simulink model "Inverse_Pendulum"  (R2025a)
settings: Solver=VariableStepAuto  StartTime=0.0  StopTime=50  RelTol=1e-3
values from neighbouring files (symbols this model uses):
  A = [ 0         0       1       0 ... (first row only)    [Inverse_Pendulum_parameters.m]    (also in Inverse_Pendulum_parameters_discrete.m; [LQG] Inverse_Pendulum_parameters.m; [LQR] Inverse_Pendulum_parameters.m)
  b = 0.00007892    (= 7.892e-05)    [Inverse_Pendulum_parameters.m]    (also in Inverse_Pendulum_parameters_discrete.m; [LQG] Inverse_Pendulum_parameters.m; [LQR] Inverse_Pendulum_parameters.m)
  B = [0;         0;          (J+m*l^2)*kt/(alp*Rm*r);        l*m*kt/(alp*Rm*r)]    [Inverse_Pendulum_parameters.m]    (also in Inverse_Pendulum_parameters_discrete.m; [LQG] Inverse_Pendulum_parameters.m; [LQR] Inverse_Pendulum_parameters.m)
  c = 0.63    [Inverse_Pendulum_parameters.m]    (also in Inverse_Pendulum_parameters_discrete.m; [LQG] Inverse_Pendulum_parameters.m; [LQR] Inverse_Pendulum_parameters.m)
  C = [1 0 0 0; 0 1 0 0]    [Inverse_Pendulum_parameters.m]    (also in Inverse_Pendulum_parameters_discrete.m; [LQG] Inverse_Pendulum_parameters.m)
  g = 9.81    [Inverse_Pendulum_parameters.m]    (also in Inverse_Pendulum_parameters_discrete.m; [LQG] Inverse_Pendulum_parameters.m; [LQR] Inverse_Pendulum_parameters.m)
  J = 0.0007176    [Inverse_Pendulum_parameters.m]    (also in Inverse_Pendulum_parameters_discrete.m = 0.000596; [LQG] Inverse_Pendulum_parameters.m; [LQR] Inverse_Pendulum_parameters.m)
  K = lqr(A,B,Q,R)    [Inverse_Pendulum_parameters.m]    (also in [LQG] Inverse_Pendulum_parameters.m; [LQR] Inverse_Pendulum_parameters.m)
  k_swing = 12    [Inverse_Pendulum_parameters.m]    (also in Inverse_Pendulum_parameters_discrete.m = 42; [LQG] Inverse_Pendulum_parameters.m; [LQR] Inverse_Pendulum_parameters.m)
  kb = 0.031    [Inverse_Pendulum_parameters.m]    (also in Inverse_Pendulum_parameters_discrete.m; [LQG] Inverse_Pendulum_parameters.m; [LQR] Inverse_Pendulum_parameters.m)
  Kk = lqe(A, G, C, Qn, Rn)    [Inverse_Pendulum_parameters.m]    (also in [LQG] Inverse_Pendulum_parameters.m)
  kt = 0.031    [Inverse_Pendulum_parameters.m]    (also in Inverse_Pendulum_parameters_discrete.m; [LQG] Inverse_Pendulum_parameters.m; [LQR] Inverse_Pendulum_parameters.m)
  l = 0.2    [Inverse_Pendulum_parameters.m]    (also in Inverse_Pendulum_parameters_discrete.m = 0.1; [LQG] Inverse_Pendulum_parameters.m; [LQR] Inverse_Pendulum_parameters.m)
  M = 0.136    [Inverse_Pendulum_parameters.m]    (also in Inverse_Pendulum_parameters_discrete.m = 0.1; [LQG] Inverse_Pendulum_parameters.m; [LQR] Inverse_Pendulum_parameters.m)
  m = 0.1    [Inverse_Pendulum_parameters.m]    (also in Inverse_Pendulum_parameters_discrete.m = 0.04467; [LQG] Inverse_Pendulum_parameters.m; [LQR] Inverse_Pendulum_parameters.m)
  r = 0.006    [Inverse_Pendulum_parameters.m]    (also in Inverse_Pendulum_parameters_discrete.m; [LQG] Inverse_Pendulum_parameters.m; [LQR] Inverse_Pendulum_parameters.m)
  Rm = 12.5    [Inverse_Pendulum_parameters.m]    (also in Inverse_Pendulum_parameters_discrete.m; [LQG] Inverse_Pendulum_parameters.m; [LQR] Inverse_Pendulum_parameters.m)
libraries: simulink x7
settings Model: Creator=ADMIN  LastModifiedBy=ADMIN
settings OptimizationCC: DefaultParameterBehavior=Inlined  EnhancedBackFolding=on  PassReuseOutputArgsAs=Individual arguments  ZeroExternalMemoryAtStartup=off  ZeroInternalMemoryAtStartup=off  OptimizeBlockOrder=speed  DifferentSizesBufferReuse=on  OptimizationCustomize=off  EfficientTunableParamExpr=on
settings DebuggingCC: ParameterTunabilityLossMsg=error
settings SFSimCC: MATLABDynamicMemAlloc=off
settings RTWCC: SystemTargetFile=ert.tlc  GenCodeOnly=on  TemplateMakefile=ert_default_tmf  Description=Embedded Coder
settings CodeAppCC: ForceParamTrailComments=on  IgnoreCustomStorageClasses=off  OperatorAnnotations=on  SimulinkDataObjDesc=on  SFDataObjDesc=on  InsertBlockDesc=on
settings ERTTargetCC: ExtModeTransport=0.0  ExtModeStaticAlloc=off  ExtModeMexFile=ext_comm  ExtModeIntrfLevel=Level1  ERTCustomFileTemplate=example_file_process.tlc  TargetLangStandard=C99 (ISO)  GenerateSampleERTMain=on

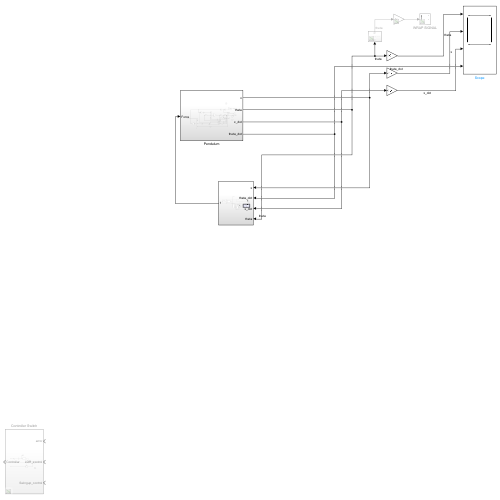
[thumbnail: Simulink's stored preview of the top-level diagram]
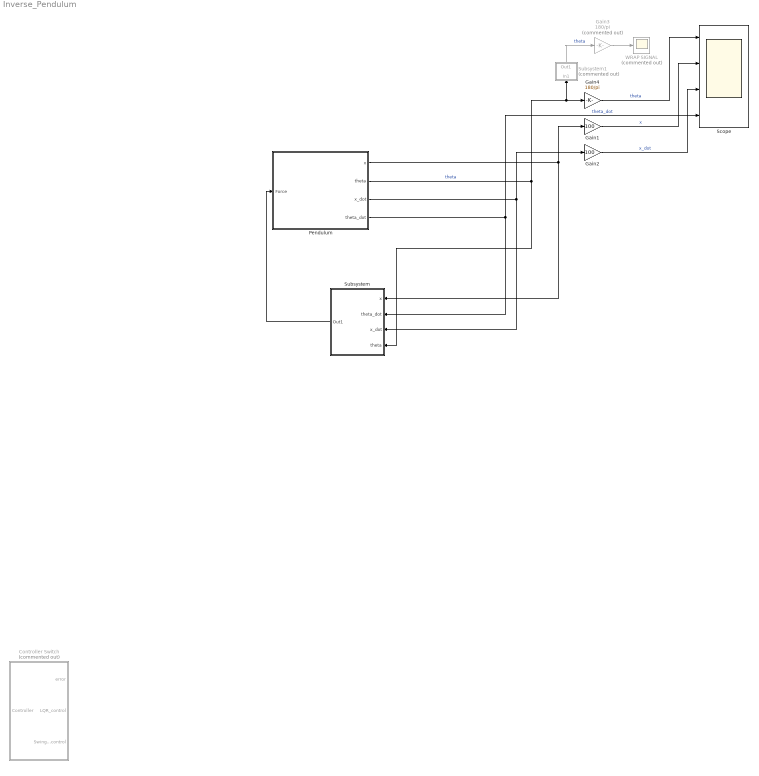
== system Inverse_Pendulum ==
  Controller Switch : Subsystem  Commented=on
  Gain1 : Gain  Gain=100
  Gain2 : Gain  Gain=100
  Gain3 : Gain  Commented=on  Gain=180/pi
  Gain4 : Gain  Gain=180/pi
  Pendulum : Subsystem
  Scope : Scope  NumInputPorts=4
      settings: ActiveDisplayYMinimum=-181.08264575614339  ActiveDisplayYMaximum=178.95893192046651
  Subsystem : Subsystem
  Subsystem1 : Subsystem  Commented=on
  WRAP SIGNAL : Scope  Commented=on
      settings: ActiveDisplayYMinimum=-145.61857492657683  ActiveDisplayYMaximum=445.48596723603623  DataLoggingVariableName=ScopeData3
  wires:
  Pendulum/1(x) -> Gain1/1, Subsystem/1(x)
  Pendulum/3(x_dot) -> Gain2/1, Subsystem/3(x_dot)
  Pendulum/4(theta_dot) -> Scope/4, Subsystem/2(theta_dot)  "theta_dot"
  Gain1/1 -> Scope/2  "x"
  Gain2/1 -> Scope/3  "x_dot"
  Pendulum/2(theta) -> Subsystem/4(theta), Subsystem1/1(In1), Gain4/1  "theta"
  Gain3/1 -> WRAP SIGNAL/1
  Subsystem1/1(Out1) -> Gain3/1  "theta"
  Gain4/1 -> Scope/1  "theta"
  Subsystem/1(Out1) -> Pendulum/1(Force)

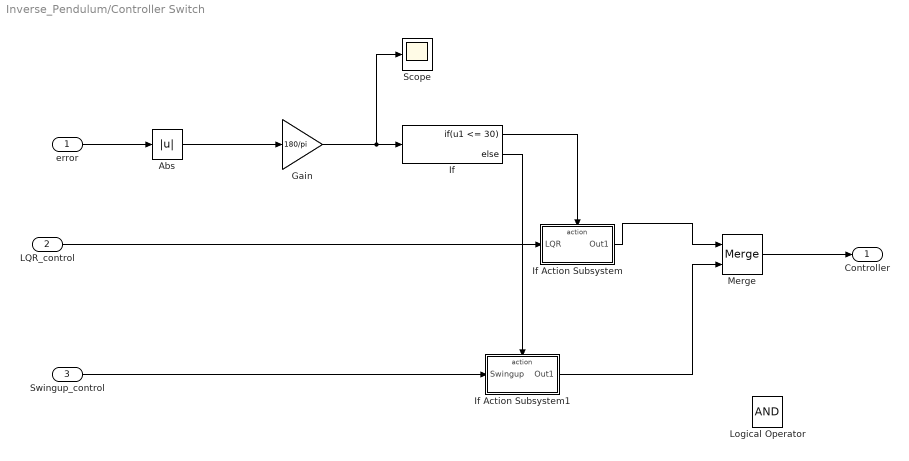
== system Inverse_Pendulum/Controller Switch ==
  error : Inport
  LQR_control : Inport  Port=2
  Swingup_control : Inport  Port=3
  Abs : Abs  SaturateOnIntegerOverflow=off
  Gain : Gain  Gain=180/pi
  If : If  IfExpression=u1 <= 30
  If Action Subsystem : Subsystem  TreatAsAtomicUnit=on
  If Action Subsystem1 : Subsystem  TreatAsAtomicUnit=on
  Logical Operator : Logic  AllPortsSameDT=off  OutDataTypeStr=boolean
  Merge : Merge
  Scope : Scope
      settings: ActiveDisplayYMinimum=-128.20702639105355  ActiveDisplayYMaximum=233.38136313352607  DataLoggingVariableName=ScopeData4
  Controller : Outport
  wires:
  error/1 -> Abs/1
  Abs/1 -> Gain/1
  Gain/1 -> Scope/1, If/1
  If/1 -> If Action Subsystem/Action
  LQR_control/1 -> If Action Subsystem/1(LQR)
  If/2 -> If Action Subsystem1/Action
  Swingup_control/1 -> If Action Subsystem1/1(Swingup)
  If Action Subsystem/1(Out1) -> Merge/1
  If Action Subsystem1/1(Out1) -> Merge/2
  Merge/1 -> Controller/1

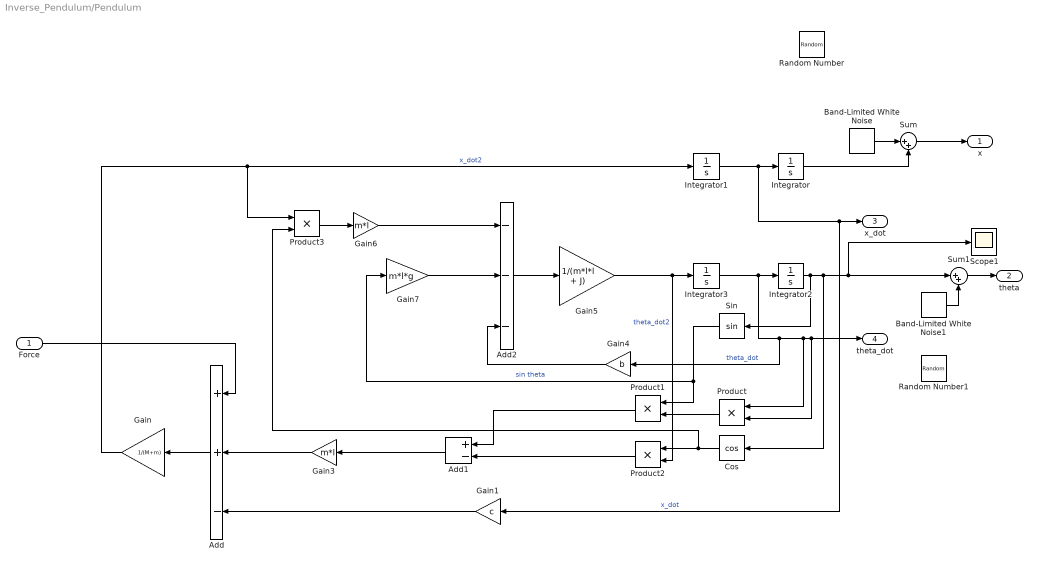
== system Inverse_Pendulum/Pendulum ==
  Force : Inport
  Add : Sum  Inputs=++-
  Add1 : Sum  Inputs=+-
  Add2 : Sum  Inputs=---
  Band-Limited White Noise : simulink/Sources/Band-Limited White Noise  Cov=[0.000001]  Ts=0.1  seed=[23341]
  Band-Limited White Noise1 : simulink/Sources/Band-Limited White Noise  Cov=[0.000001]  Ts=0.1  seed=[23341]
  Cos : Trigonometry  Operator=cos
  Gain : Gain  Gain=1/(M+m)
  Gain1 : Gain  Gain=c
  Gain3 : Gain  Gain=m*l
  Gain4 : Gain  Gain=b
  Gain5 : Gain  Gain=1/(m*l*l + J)
  Gain6 : Gain  Gain=m*l
  Gain7 : Gain  Gain=m*l*g
  Integrator{,1..3} (4 alike) : Integrator
  Product{,1..3} (4 alike) : Product
  Random Number : RandomNumber  Variance=0.001  SampleTime=0.1
  Random Number1 : RandomNumber  Variance=0.0001  SampleTime=0.1
  Scope1 : Scope
      settings: ActiveDisplayYMinimum=-24.198967580601451  ActiveDisplayYMaximum=45.388514798043275  DataLoggingVariableName=ScopeData2
  Sin : Trigonometry
  Sum : Sum  Inputs=|++
  Sum1 : Sum  Inputs=|++
  x : Outport
  theta : Outport  Port=2
  x_dot : Outport  Port=3
  theta_dot : Outport  Port=4
  wires:
  Gain3/1 -> Add/2
  Integrator/1 -> Sum/2
  Integrator1/1 -> Gain1/1, x_dot/1, Integrator/1  "x_dot"
  Product/1 -> Product1/2
  Force/1 -> Add/1
  Product1/1 -> Add1/1
  Sin/1 -> Gain7/1, Product1/1  "sin theta"
  Gain6/1 -> Add2/1
  Add2/1 -> Gain5/1
  Integrator3/1 -> theta_dot/1, Product/2, Product/1, Gain4/1, Integrator2/1  "theta_dot"
  Gain5/1 -> Product2/2, Integrator3/1  "theta_dot2"
  Integrator2/1 -> Cos/1, Sum1/1, Scope1/1, Sin/1
  Add/1 -> Gain/1
  Gain/1 -> Product3/1, Integrator1/1  "x_dot2"
  Gain7/1 -> Add2/2
  Cos/1 -> Product3/2, Product2/1
  Product3/1 -> Gain6/1
  Gain4/1 -> Add2/3
  Product2/1 -> Add1/2
  Add1/1 -> Gain3/1
  Gain1/1 -> Add/3
  Sum/1 -> x/1
  Sum1/1 -> theta/1
  Band-Limited White Noise/1 -> Sum/1
  Band-Limited White Noise1/1 -> Sum1/2

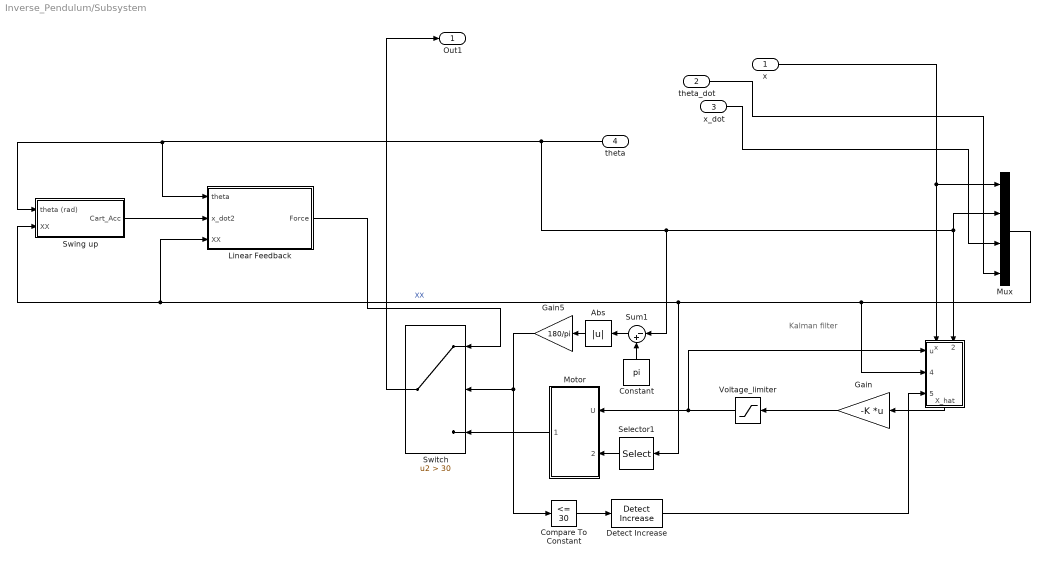
== system Inverse_Pendulum/Subsystem ==
  note: Kalman filter
  x : Inport
  theta_dot : Inport  Port=2
  x_dot : Inport  Port=3
  theta : Inport  Port=4
  " " : Subsystem
      settings: PortSchema="{\"entries\":[{\"content\":{\"sides\":[{\"content\":{\"connectorIds\":[\"In1\",\"In2\"]},\"type\":\"ConnectorPlacement.EquallySpacedRectSide\",\"uuid\":\"213b765e-47fa-44cf-837a-76b4f9098c24\"},{\"content\":{\"connectorIds\":[\"Out1\"],\"side\":\"RIGHT\"},\"type\":\"ConnectorPlacement.EquallySpacedRectSide\",\"uuid\":\"45a7b12b-a4ed-4c45-ac3d-ce2c11d0f41c\"},{\"content\":{\"connectorIds\":[\"In3\",\"In4\",\"In5\"],\"side\":\"TOP\"},\"type\":\"ConnectorPlacement.EquallySpacedRectSide\",\"uuid\":\"3cd53e22-245a-4d13-9dac-306e9bf70ac5\"}]},\"type\":\"ConnectorPlacement.EquallySpacedConnector\",\"uuid\":\"c2a62d5e-615a-4291-9189-bd7e79077aeb\"}],\"packageUris\":[\"http://schema.mathworks.com/mf0/Connector/R2020b\"],\"version\":\"1.0\"}"
  Abs : Abs  SaturateOnIntegerOverflow=off
  Compare To Constant : simulink/Logic and Bit Operations/Compare To Constant  relop=<=  const=30  OutDataTypeStr=boolean
  Constant : Constant  Value=pi
  Detect Increase : simulink/Logic and Bit Operations/Detect Increase  vinit=0.0  OutDataTypeStr=boolean
  Gain : Gain  Gain=-K  Multiplication=Matrix(K*u)
  Gain5 : Gain  Gain=180/pi
  Linear Feedback : Subsystem
  Motor : Subsystem
  Mux : Mux
  Selector1 : Selector  InputPortWidth=4  IndexOptions=Index vector (dialog)  Indices=3  OutputSizes=1
  Sum1 : Sum  Inputs=|-+
  "Swing up " : Subsystem
  Switch : Switch  Criteria=u2 > Threshold  Threshold=30  SaturateOnIntegerOverflow=off  InputSameDT=off
  Voltage_limiter : Saturate  UpperLimit=12  LowerLimit=-12
  Out1 : Outport
  wires:
  Detect Increase/1 -> " "/5(Rising)
  theta/1 -> Mux/2, " "/2(theta), Sum1/1, "Swing up "/1(theta (rad)), Linear Feedback/1(theta)
  Gain/1 -> Voltage_limiter/1
  " "/1(X_hat) -> Gain/1
  Voltage_limiter/1 -> Motor/1(U), " "/3(u)
  x/1 -> Mux/1, " "/1(x)
  Selector1/1 -> Motor/2(x_dot)
  Compare To Constant/1 -> Detect Increase/1
  "Swing up "/1(Cart_Acc) -> Linear Feedback/2(x_dot2)
  Constant/1 -> Sum1/2
  Sum1/1 -> Abs/1
  Gain5/1 -> Compare To Constant/1, Switch/2
  Linear Feedback/1(Force) -> Switch/1
  Mux/1 -> Selector1/1, "Swing up "/2(XX), Linear Feedback/3(XX), " "/4(State)  "XX"
  Motor/1(Force) -> Switch/3
  Abs/1 -> Gain5/1
  Switch/1 -> Out1/1
  theta_dot/1 -> Mux/4
  x_dot/1 -> Mux/3

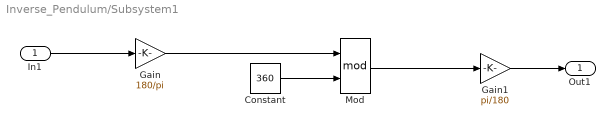
== system Inverse_Pendulum/Subsystem1 ==
  In1 : Inport
  Constant : Constant  Value=360
  Gain : Gain  Gain=180/pi
  Gain1 : Gain  Gain=pi/180
  Mod : Math  Operator=mod
  Out1 : Outport
  wires:
  In1/1 -> Gain/1
  Constant/1 -> Mod/2
  Gain/1 -> Mod/1
  Mod/1 -> Gain1/1
  Gain1/1 -> Out1/1

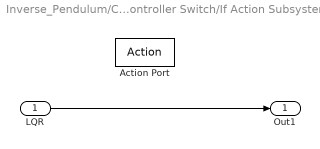
== system Inverse_Pendulum/Controller Switch/If Action Subsystem ==
  LQR : Inport
  Action Port : ActionPort  ActionPortLabel=if(u1 <= 30)
  Out1 : Outport
  wires:
  LQR/1 -> Out1/1

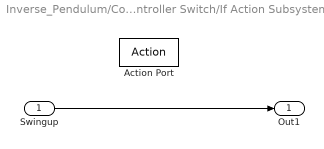
== system Inverse_Pendulum/Controller Switch/If Action Subsystem1 ==
  Swingup : Inport
  Action Port : ActionPort  ActionPortLabel=else
  Out1 : Outport
  wires:
  Swingup/1 -> Out1/1

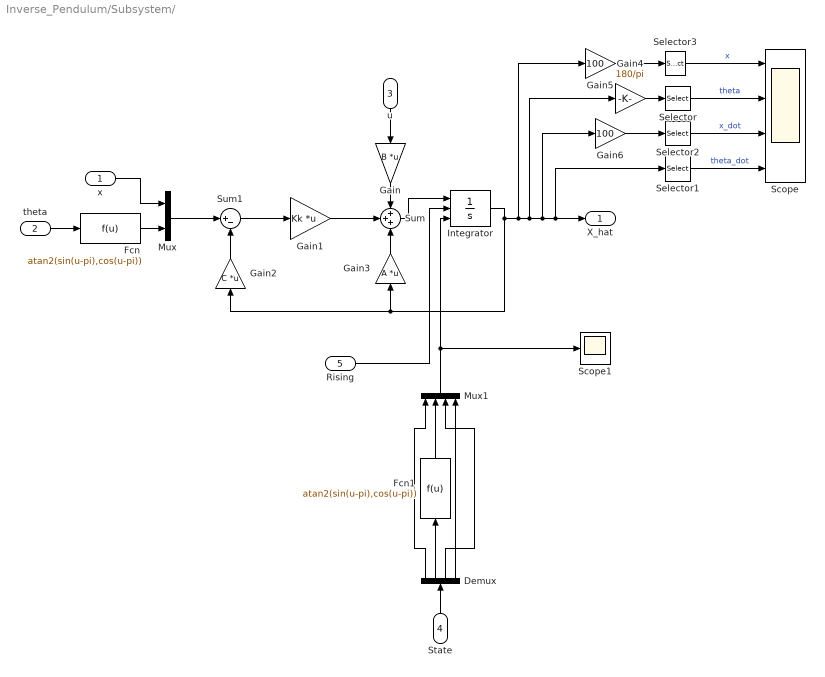
== system Inverse_Pendulum/Subsystem/  ==
  x : Inport
  theta : Inport  Port=2
  u : Inport  Port=3
  State : Inport  Port=4
  Rising : Inport  Port=5
  Demux : Demux
  Fcn : Fcn  Expr=atan2(sin(u-pi),cos(u-pi))
  Fcn1 : Fcn  Expr=atan2(sin(u-pi),cos(u-pi))
  Gain : Gain  Gain=B  Multiplication=Matrix(K*u)
  Gain1 : Gain  Gain=Kk  Multiplication=Matrix(K*u)
  Gain2 : Gain  Gain=C  Multiplication=Matrix(K*u)
  Gain3 : Gain  Gain=A  Multiplication=Matrix(K*u)
  Gain4 : Gain  Gain=180/pi
  Gain5 : Gain  Gain=100
  Gain6 : Gain  Gain=100
  Integrator : Integrator  ExternalReset=rising  InitialConditionSource=external
  Mux : Mux  Inputs=2
  Mux1 : Mux
  Scope : Scope  NumInputPorts=4
      settings: ActiveDisplayYMinimum=-342.5574840436575  ActiveDisplayYMaximum=141.24899425477486  DataLoggingVariableName=ScopeData5
  Scope1 : Scope
      settings: ActiveDisplayYMinimum=-8.0230697293546722  ActiveDisplayYMaximum=13.271729731553696
  Selector : Selector  InputPortWidth=4  IndexOptions=Index vector (dialog)  Indices=2  OutputSizes=1
  Selector1 : Selector  InputPortWidth=4  IndexOptions=Index vector (dialog)  Indices=4  OutputSizes=1
  Selector2 : Selector  InputPortWidth=4  IndexOptions=Index vector (dialog)  Indices=3  OutputSizes=1
  Selector3 : Selector  InputPortWidth=4  IndexOptions=Index vector (dialog)  Indices=1  OutputSizes=1
  Sum : Sum  Inputs=+++
  Sum1 : Sum  Inputs=|+-
  X_hat : Outport
  wires:
  x/1 -> Mux/1
  Gain/1 -> Sum/1
  Sum1/1 -> Gain1/1
  Gain2/1 -> Sum1/2
  Gain1/1 -> Sum/2
  Gain3/1 -> Sum/3
  Sum/1 -> Integrator/1
  Integrator/1 -> Gain2/1, Gain3/1, Gain5/1, Gain4/1, Gain6/1, Selector1/1, X_hat/1
  u/1 -> Gain/1
  Mux/1 -> Sum1/1
  Selector/1 -> Scope/2  "theta"
  Selector1/1 -> Scope/4  "theta_dot"
  Selector2/1 -> Scope/3  "x_dot"
  Selector3/1 -> Scope/1  "x"
  Gain4/1 -> Selector/1
  Gain5/1 -> Selector3/1
  Gain6/1 -> Selector2/1
  theta/1 -> Fcn/1
  Fcn/1 -> Mux/2
  Rising/1 -> Integrator/2
  State/1 -> Demux/1
  Demux/2 -> Fcn1/1
  Fcn1/1 -> Mux1/2
  Demux/1 -> Mux1/1
  Demux/3 -> Mux1/3
  Demux/4 -> Mux1/4
  Mux1/1 -> Scope1/1, Integrator/3

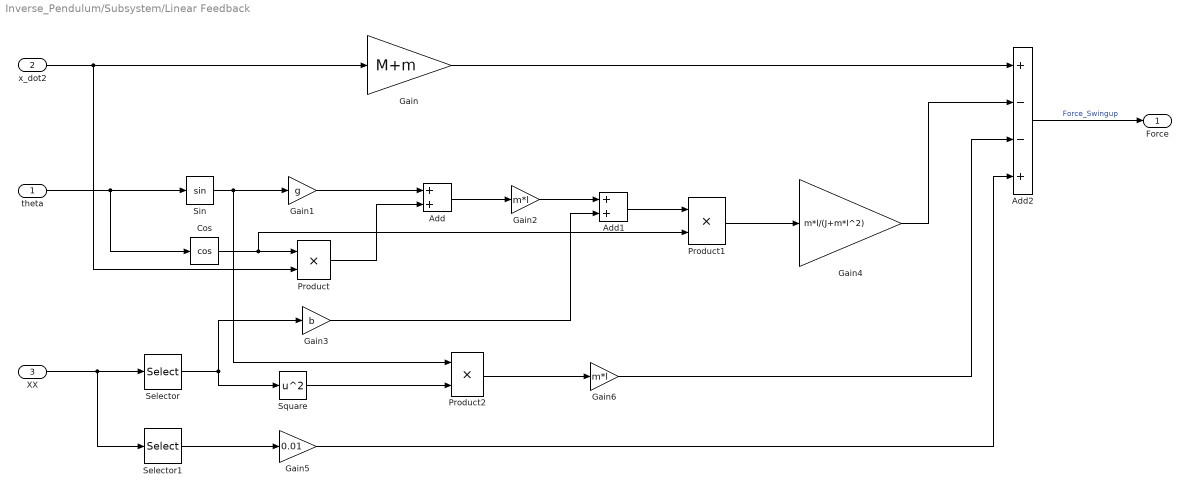
== system Inverse_Pendulum/Subsystem/Linear Feedback ==
  theta : Inport
  x_dot2 : Inport  Port=2
  XX : Inport  Port=3
  Add : Sum
  Add1 : Sum
  Add2 : Sum  Inputs=+--+
  Cos : Trigonometry  Operator=cos
  Gain : Gain  Gain=M+m
  Gain1 : Gain  Gain=g
  Gain2 : Gain  Gain=m*l
  Gain3 : Gain  Gain=b
  Gain4 : Gain  Gain=m*l/(J+m*l^2)
  Gain5 : Gain  Gain=0.01
  Gain6 : Gain  Gain=m*l
  Product : Product
  Product1 : Product
  Product2 : Product
  Selector : Selector  InputPortWidth=4  IndexOptions=Index vector (dialog)  Indices=4  OutputSizes=1
  Selector1 : Selector  InputPortWidth=4  IndexOptions=Index vector (dialog)  Indices=3  OutputSizes=1
  Sin : Trigonometry
  Square : Math  Operator=square
  Force : Outport
  wires:
  theta/1 -> Cos/1, Sin/1
  x_dot2/1 -> Product/2, Gain/1
  Cos/1 -> Product1/2, Product/1
  Sin/1 -> Product2/1, Gain1/1
  Gain1/1 -> Add/1
  Product/1 -> Add/2
  Add/1 -> Gain2/1
  XX/1 -> Selector1/1, Selector/1
  Selector/1 -> Gain3/1, Square/1
  Gain2/1 -> Add1/1
  Gain3/1 -> Add1/2
  Add1/1 -> Product1/1
  Product1/1 -> Gain4/1
  Square/1 -> Product2/2
  Selector1/1 -> Gain5/1
  Product2/1 -> Gain6/1
  Gain6/1 -> Add2/3
  Gain4/1 -> Add2/2
  Gain/1 -> Add2/1
  Gain5/1 -> Add2/4
  Add2/1 -> Force/1  "Force_Swingup"

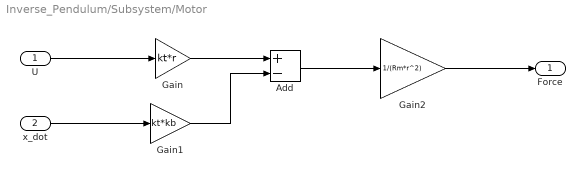
== system Inverse_Pendulum/Subsystem/Motor ==
  U : Inport
  x_dot : Inport  Port=2
  Add : Sum  Inputs=+-
  Gain : Gain  Gain=kt*r
  Gain1 : Gain  Gain=kt*kb
  Gain2 : Gain  Gain=1/(Rm*r^2)
  Force : Outport
  wires:
  U/1 -> Gain/1
  x_dot/1 -> Gain1/1
  Gain/1 -> Add/1
  Gain1/1 -> Add/2
  Add/1 -> Gain2/1
  Gain2/1 -> Force/1

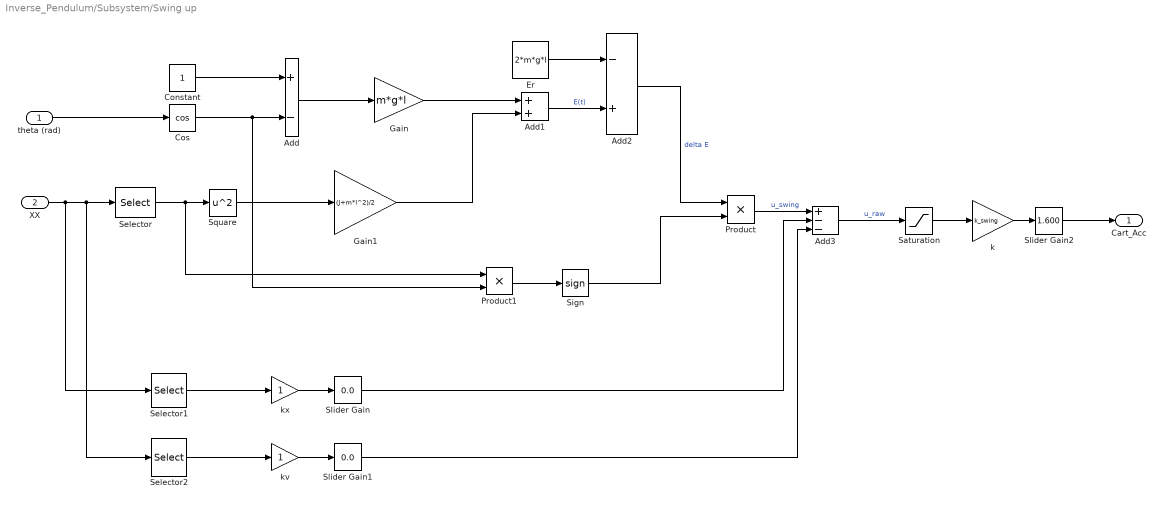
== system Inverse_Pendulum/Subsystem/Swing up  ==
  theta (rad) : Inport
  XX : Inport  Port=2
  Add : Sum  Inputs=+-
  Add1 : Sum
  Add2 : Sum  Inputs=-+
  Add3 : Sum  Inputs=+--
  Constant : Constant
  Cos : Trigonometry  Operator=cos
  Er : Constant  Value=2*m*g*l
  Gain : Gain  Gain=m*g*l
  Gain1 : Gain  Gain=(J+m*l^2)/2
  Product : Product
  Product1 : Product
  Saturation : Saturate  UpperLimit=3*g  LowerLimit=-3*g
  Selector : Selector  InputPortWidth=4  IndexOptions=Index vector (dialog)  Indices=4  OutputSizes=1
  Selector1 : Selector  InputPortWidth=4  IndexOptions=Index vector (dialog)  Indices=1  OutputSizes=1
  Selector2 : Selector  InputPortWidth=4  IndexOptions=Index vector (dialog)  Indices=2  OutputSizes=1
  Sign : Signum
  Slider Gain : simulink/Math Operations/Slider Gain  gain=0.0  low=0  high=2
  Slider Gain1 : simulink/Math Operations/Slider Gain  gain=0.0  low=0  high=2
  Slider Gain2 : simulink/Math Operations/Slider Gain  gain=1.600  low=0  high=2
  Square : Math  Operator=square
  k : Gain  Gain=k_swing
  kv : Gain
  kx : Gain
  Cart_Acc : Outport
  wires:
  theta (rad)/1 -> Cos/1
  Cos/1 -> Product1/2, Add/2
  Constant/1 -> Add/1
  Add/1 -> Gain/1
  XX/1 -> Selector1/1, Selector2/1, Selector/1
  Selector/1 -> Product1/1, Square/1
  Gain/1 -> Add1/1
  Square/1 -> Gain1/1
  Gain1/1 -> Add1/2
  Add1/1 -> Add2/2  "E(t)"
  Er/1 -> Add2/1
  Add2/1 -> Product/1  "delta E"
  Sign/1 -> Product/2
  Product1/1 -> Sign/1
  Product/1 -> Add3/1  "u_swing"
  Slider Gain/1 -> Add3/2
  Selector1/1 -> kx/1
  kx/1 -> Slider Gain/1
  Selector2/1 -> kv/1
  kv/1 -> Slider Gain1/1
  Slider Gain1/1 -> Add3/3
  Add3/1 -> Saturation/1  "u_raw"
  k/1 -> Slider Gain2/1
  Slider Gain2/1 -> Cart_Acc/1
  Saturation/1 -> k/1
